simulink model "TorqueControl_QuadRad_FF_SMC"  (R2014a)
settings: Solver=ode4  StartTime=0.0  StopTime=4500  FixedStep=1  MaxStep=1  MinStep=0.1  RelTol=1e-3
undefined symbols (not defined in the file): bike, cont, param, paramIH, rider, route, sigbuilder_block
libraries: simulink x1, aerolibconvert2 x1
settings Model: Creator=Daniel  LastModifiedBy=meyer
settings SolverCC: InitialStep=1

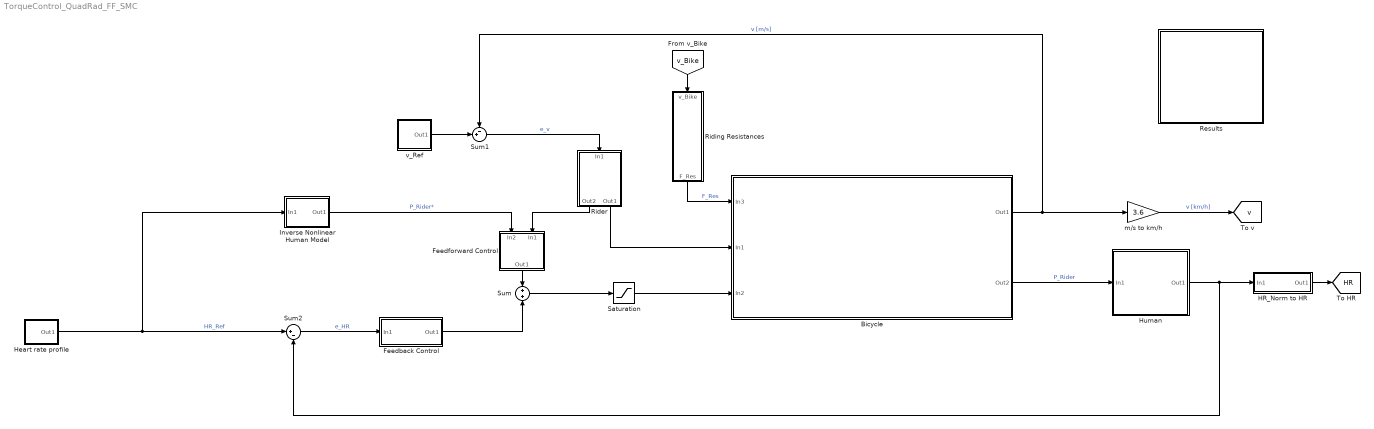
== system TorqueControl_QuadRad_FF_SMC ==
  Bicycle : Subsystem  mask(Bicycle Dynamics){}
      mask help:
      | Calculates the speed of the bicycle based on the propulsion forces of motor
      | bicycle rider against the resistance forces of the environment.
      mask Display:
      | port_label('input',1,'F_Res [N]')
      | port_label('input',2,'F_Rider [N]')
      | port_label('input',3,'T_M_ref')
      | port_label('output',1,'v_Bike [m/s]')
      | port_label('output',2,'P_Rider [W]')
      | image('QuadRad.jpg', [100 20 185 160])
  Feedback Control : Subsystem
  Feedforward Control : Subsystem
  HR_Norm to HR : Subsystem
  Heart rate profile : Subsystem
  Human : Subsystem
  Inverse Nonlinear Human Model : Subsystem
  Results : Subsystem
  Rider : Subsystem
  Riding Resistances : Subsystem
  Saturation : Saturate  UpperLimit=bike.motor.T_max  LowerLimit=bike.motor.T_min  ZeroCross=off
  Sum : Sum  Inputs=+|+
  Sum1 : Sum  Inputs=-+|
  Sum2 : Sum  Inputs=|+-
  m/s to km/h : Gain  Gain=3.6
  v_Ref : Subsystem
  tag scope: HR=global, v=global
  wires:
  Bicycle/1(Out1) -> Sum1/1, m/s to km/h/1  "v [m/s]"
  Riding Resistances/1(F_Res) -> Bicycle/1(In3)  "F_Res"
  m/s to km/h/1 -> [v]  "v [km/h]"
  [v_Bike] -> Riding Resistances/1(v_Bike)
  Sum1/1 -> Rider/1(In1)  "e_v"
  Rider/2(Out1) -> Bicycle/2(In1)
  HR_Norm to HR/1(Out1) -> [HR]
  Human/1(Out1) -> HR_Norm to HR/1(In1), Sum2/2
  Bicycle/2(Out2) -> Human/1(In1)  "P_Rider"
  Sum2/1 -> Feedback Control/1(In1)  "e_HR"
  Heart rate profile/1(Out1) -> Inverse Nonlinear Human Model/1(In1), Sum2/1  "HR_Ref"
  v_Ref/1(Out1) -> Sum1/2
  Feedback Control/1(Out1) -> Sum/2
  Sum/1 -> Saturation/1
  Rider/1(Out2) -> Feedforward Control/2(In1)
  Inverse Nonlinear Human Model/1(Out1) -> Feedforward Control/1(In2)  "P_Rider*"
  Feedforward Control/1(Out1) -> Sum/1
  Saturation/1 -> Bicycle/3(In2)

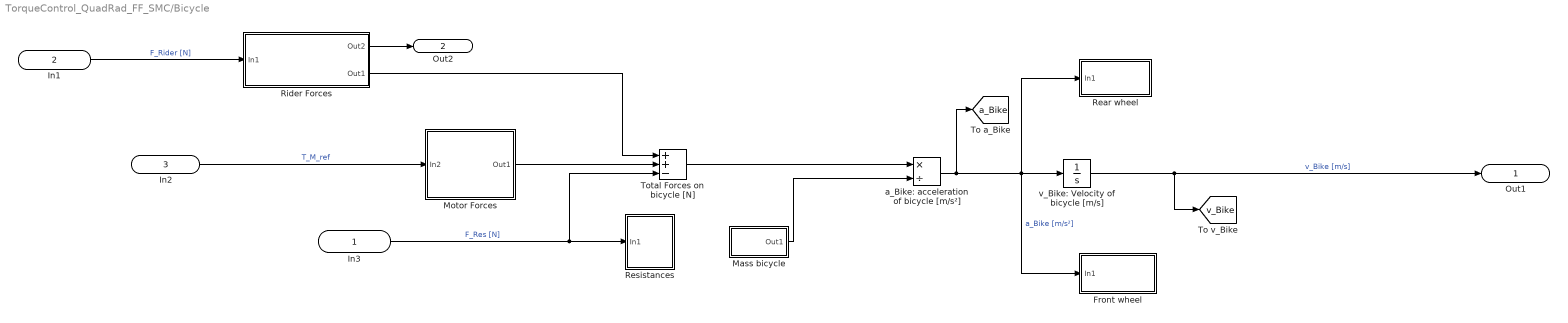
== system TorqueControl_QuadRad_FF_SMC/Bicycle ==
  In3 : Inport
  In1 : Inport  Port=2
  In2 : Inport  Port=3
  Front wheel : Subsystem
  Mass bicycle : Subsystem
  Motor Forces : Subsystem
  Rear wheel : Subsystem
  Resistances : Subsystem
  Rider Forces : Subsystem
  Total Forces on bicycle [N] : Sum  Inputs=++-
  a_Bike: acceleration of bicycle [m/s²] : Product  Inputs=*/
  v_Bike: Velocity of bicycle [m/s] : Integrator
  Out1 : Outport
  Out2 : Outport  Port=2
  tag scope: a_Bike=global, v_Bike=global
  wires:
  Mass bicycle/1(Out1) -> a_Bike: acceleration of bicycle [m/s²]/2
  Motor Forces/1(Out1) -> Total Forces on bicycle [N]/2
  In2/1 -> Motor Forces/1(In2)  "T_M_ref"
  Rider Forces/2(Out1) -> Total Forces on bicycle [N]/1
  Rider Forces/1(Out2) -> Out2/1
  In1/1 -> Rider Forces/1(In1)  "F_Rider [N]"
  a_Bike: acceleration of bicycle [m/s²]/1 -> v_Bike: Velocity of bicycle [m/s]/1, Rear wheel/1(In1), Front wheel/1(In1), [a_Bike]  "a_Bike [m/s²]"
  v_Bike: Velocity of bicycle [m/s]/1 -> Out1/1, [v_Bike]  "v_Bike [m/s]"
  Total Forces on bicycle [N]/1 -> a_Bike: acceleration of bicycle [m/s²]/1
  In3/1 -> Total Forces on bicycle [N]/3, Resistances/1(In1)  "F_Res [N]"

== system TorqueControl_QuadRad_FF_SMC/Feedback Control ==
  In1 : Inport
  Constant : Constant  Value=cont.c
  Derivative : Derivative
  Multiport Switch : MultiPortSwitch  Inputs=2
  Quasi-1-SMC : Subsystem
  Saturation : Saturate  UpperLimit=cont.upLim  LowerLimit=cont.lowLim
  Simple-1-SMC : Subsystem
  Out1 : Outport
  tag scope: T_M_FB=global, e=global, e_dot=global
  wires:
  Derivative/1 -> [e_dot]
  Quasi-1-SMC/1(Out1) -> Multiport Switch/3
  Simple-1-SMC/1(Out1) -> Multiport Switch/2
  Constant/1 -> Multiport Switch/1
  Saturation/1 -> [T_M_FB], Out1/1  "T_M_FB"
  In1/1 -> Simple-1-SMC/1(In1), Quasi-1-SMC/1(In1), [e], Derivative/1  "e_HR"
  Multiport Switch/1 -> Saturation/1  "T_M_FB"

== system TorqueControl_QuadRad_FF_SMC/Feedforward Control ==
  In2 : Inport
  In1 : Inport  Port=2
  Feedforward Control : Subsystem
  Sum3 : Sum  Inputs=-|+
  Out1 : Outport
  tag scope: T_M_FF=global
  wires:
  Feedforward Control/1(Out1) -> Sum3/1
  In2/1 -> Feedforward Control/1(In1)  "P_R*"
  In1/1 -> Sum3/2  "T_R"
  Sum3/1 -> Out1/1, [T_M_FF]  "T_M_FF"

== system TorqueControl_QuadRad_FF_SMC/HR_Norm to HR ==
  In1 : Inport
  Add : Sum
  HR_Rest : Constant  Value=rider.HR_rest
  HR_max : Constant  Value=rider.HR_max
  Product : Product
  Out1 : Outport
  wires:
  HR_max/1 -> Product/2
  Add/1 -> Out1/1  "HR"
  Product/1 -> Add/1
  In1/1 -> Product/1  "HR_Norm"
  HR_Rest/1 -> Add/2

== system TorqueControl_QuadRad_FF_SMC/Heart rate profile ==
  Choose HR_Profile : Constant  Value=3
  Constant : Constant  Value=140
  From Workspace : FromWorkspace  VariableName=HRPROFILE  SampleTime=0
  HR to HR_Norm : Subsystem
  Multiport Switch : MultiPortSwitch
  Signal Builder : Subsystem  Tag=STV Subsys  LoadFcn=sigbuilder_block('load');  StartFcn=sigbuilder_block('start');  StopFcn=sigbuilder_block('stop');  ClipboardFcn=sigbuilder_block('clipboard');  mask(Sigbuilder block){}
      mask help: Simulink:masks:SigbuilderBlock_MD
      mask init:
      | if ~strcmp(get_param(bdroot(gcbh),'SimulationStatus'),'stopped') tuvar = sigbuilder_block('maskInit'); end
      settings: CopyFcn=sigbuilder_block('copy');  DeleteFcn=sigbuilder_block('delete');  ModelCloseFcn=sigbuilder_block('modelClose');  PreSaveFcn=sigbuilder_block('preSave');  PauseFcn=sigbuilder_block('pause');  ContinueFcn=sigbuilder_block('continue');  NameChangeFcn=sigbuilder_block('namechange');  OpenFcn=sigbuilder_block('open',[216 88.5 550.5 394.5 ]);  CloseFcn=sigbuilder_block('close');
      mask Display: plot(0, 0, 100, 100,[2, 2, 32, 32, 2], [68, 8, 8, 68, 68],[32, 2], [38, 38], [32, 19, 2],[53, 60, 44], [32, 17, 17, 2],[16, 16, 31, 31]);txt = getActiveGroup(gcbh);text(2, 100, txt,'verticalAlignment', 'top');
  Out1 : Outport
  tag scope: HR_Ref=global, HR_Ref_Norm=global
  wires:
  Multiport Switch/1 -> HR to HR_Norm/1(In1), [HR_Ref]  "HRRef"
  HR to HR_Norm/1(Out1) -> [HR_Ref_Norm], Out1/1  "HR_Ref"
  Signal Builder/1(Signal 1) -> Multiport Switch/3  "HRRef"
  Constant/1 -> Multiport Switch/2
  Choose HR_Profile/1 -> Multiport Switch/1
  From Workspace/1 -> Multiport Switch/4

== system TorqueControl_QuadRad_FF_SMC/Human ==
  In1 : Inport
  Nonlinear Human Model : Subsystem
  Power to Power_Norm : Subsystem
  Scopex2 : Scope
      settings: SaveName=ScopeData2
  Out1 : Outport
  tag scope: x1=global, x2=global
  wires:
  In1/1 -> Power to Power_Norm/1(In1)  "P_Rider"
  Nonlinear Human Model/1(Out1) -> [x1], Out1/1  "Heart rate"
  Nonlinear Human Model/2(Out2) -> [x2], Scopex2/1
  Power to Power_Norm/1(Out1) -> Nonlinear Human Model/1(In1)

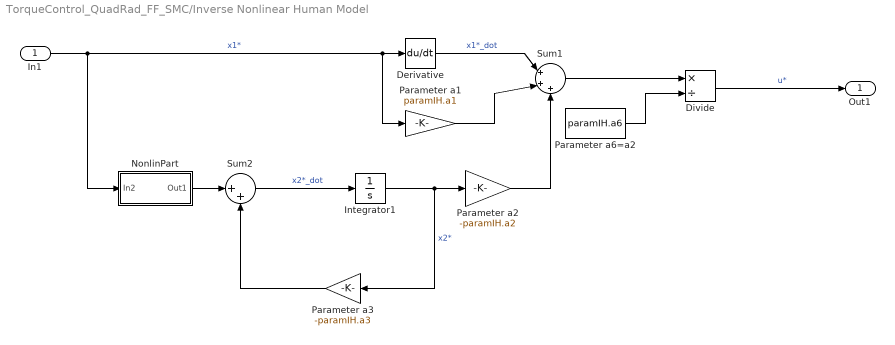
== system TorqueControl_QuadRad_FF_SMC/Inverse Nonlinear Human Model ==
  In1 : Inport
  Derivative : Derivative
  Divide : Product  Inputs=*/
  Integrator1 : Integrator
  NonlinPart : Subsystem
  Parameter a1 : Gain  Gain=paramIH.a1
  Parameter a2 : Gain  Gain=-paramIH.a2
  Parameter a3 : Gain  Gain=-paramIH.a3
  Parameter a6=a2 : Constant  Value=paramIH.a6
  Sum1 : Sum  Inputs=|+++
  Sum2 : Sum  Inputs=|++
  Out1 : Outport
  wires:
  Parameter a2/1 -> Sum1/3
  In1/1 -> Parameter a1/1, Derivative/1, NonlinPart/1(In2)  "x1*"
  Parameter a3/1 -> Sum2/2
  Sum2/1 -> Integrator1/1  "x2*_dot"
  Derivative/1 -> Sum1/1  "x1*_dot"
  Parameter a1/1 -> Sum1/2
  Sum1/1 -> Divide/1
  Parameter a6=a2/1 -> Divide/2
  Divide/1 -> Out1/1  "u*"
  NonlinPart/1(Out1) -> Sum2/1
  Integrator1/1 -> Parameter a3/1, Parameter a2/1  "x2*"

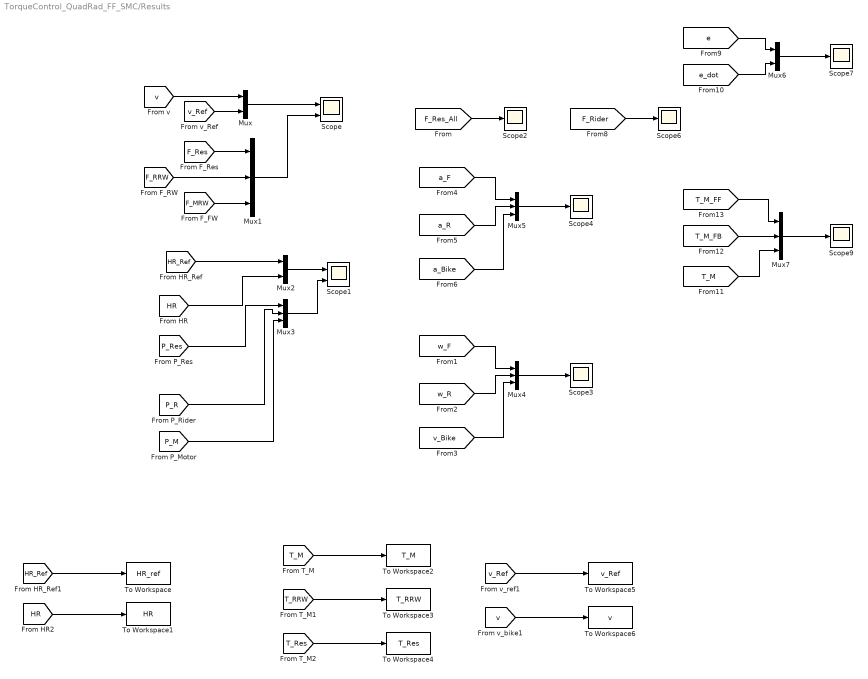
== system TorqueControl_QuadRad_FF_SMC/Results ==
  Mux : Mux  Inputs=2
  Mux{1,3..5,7} (5 alike) : Mux  Inputs=3
  Mux2 : Mux  Inputs=2
  Mux6 : Mux  Inputs=2
  Scope : Scope  NumInputPorts=2
      settings: TimeRange=4500  YMin=0~-50  YMax=25~200
  Scope1 : Scope  NumInputPorts=2
      settings: TimeRange=4500  YMin=75~0  YMax=155~375
  Scope{2..4,6..7,9} (6 alike) : Scope
      Scope2 settings: SaveName=ScopeData3
      Scope3 settings: SaveName=ScopeData4
      Scope4 settings: SaveName=ScopeData5
      Scope6 settings: SaveName=ScopeData7
      Scope7 settings: SaveName=ScopeData8
      Scope9 settings: SaveName=ScopeData10
  To Workspace : ToWorkspace  VariableName=HR_ref  SaveFormat=Timeseries  SampleTime=-1
  To Workspace1 : ToWorkspace  VariableName=HR  SaveFormat=Timeseries  SampleTime=-1
  To Workspace2 : ToWorkspace  VariableName=T_M  SaveFormat=Timeseries  SampleTime=-1
  To Workspace3 : ToWorkspace  VariableName=T_RRW  SaveFormat=Timeseries  SampleTime=-1
  To Workspace4 : ToWorkspace  VariableName=T_Res  SaveFormat=Timeseries  SampleTime=-1
  To Workspace5 : ToWorkspace  VariableName=v_Ref  SaveFormat=Timeseries  SampleTime=-1
  To Workspace6 : ToWorkspace  VariableName=v  SaveFormat=Timeseries  SampleTime=-1
  wires:
  [v] -> Mux/1
  [v_Ref] -> Mux/2
  Mux/1 -> Scope/1
  [F_Res] -> Mux1/1
  [F_MRW] -> Mux1/3
  Mux1/1 -> Scope/2
  [F_RRW] -> Mux1/2
  [HR_Ref] -> Mux2/1
  [HR] -> Mux2/2
  Mux2/1 -> Scope1/1
  [P_R] -> Mux3/2
  Mux3/1 -> Scope1/2
  [P_M] -> Mux3/3
  [P_Res] -> Mux3/1
  [F_Res_All] -> Scope2/1
  [w_F] -> Mux4/1
  [w_R] -> Mux4/2
  [v_Bike] -> Mux4/3
  Mux4/1 -> Scope3/1
  [a_F] -> Mux5/1
  [a_R] -> Mux5/2
  [a_Bike] -> Mux5/3
  Mux5/1 -> Scope4/1
  [F_Rider] -> Scope6/1
  Mux6/1 -> Scope7/1
  [e] -> Mux6/1
  [e_dot] -> Mux6/2
  [T_M] -> Mux7/3
  Mux7/1 -> Scope9/1
  [T_M_FF] -> Mux7/1
  [T_M_FB] -> Mux7/2
  [HR_Ref] -> To Workspace/1
  [HR] -> To Workspace1/1
  [T_M] -> To Workspace2/1
  [T_RRW] -> To Workspace3/1
  [T_Res] -> To Workspace4/1
  [v_Ref] -> To Workspace5/1
  [v] -> To Workspace6/1

== system TorqueControl_QuadRad_FF_SMC/Rider ==
  In1 : Inport
  Human Con : simulink/Continuous/PID Controller  Controller=PID  TimeDomain=Continuous-time  SampleTime=1  IntegratorMethod=Forward Euler  FilterMethod=Forward Euler  Form=Parallel  P=100  I=10  D=0  N=0  InitialConditionSource=internal  InitialConditionForIntegrator=0  InitialConditionForFilter=0  ExternalReset=none  LimitOutput=on  UpperSaturationLimit=900  LowerSaturationLimit=0  LinearizeAsGain=on  AntiWindupMode=none  Kb=1  TrackingMode=off  Kt=1  PParamMin=[]  PParamMax=[]  IParamMin=[]  IParamMax=[]  DParamMin=[]  DParamMax=[]  NParamMin=[]  NParamMax=[]  KbParamMin=[]  KbParamMax=[]  KtParamMin=[]  KtParamMax=[]  POutMin=[]  POutMax=[]  IOutMin=[]  IOutMax=[]  DOutMin=[]  DOutMax=[]  NOutMin=[]  NOutMax=[]  KbOutMin=[]  KbOutMax=[]  KtOutMin=[]  KtOutMax=[]  IntegratorOutMin=[]  IntegratorOutMax=[]  FilterOutMin=[]  FilterOutMax=[]  SumOutMin=[]  SumOutMax=[]  SumI1OutMin=[]  SumI1OutMax=[]  SumI2OutMin=[]  SumI2OutMax=[]  SumI3OutMin=[]  SumI3OutMax=[]  SumDOutMin=[]  SumDOutMax=[]  SaturationOutMin=[]  SaturationOutMax=[]  IntegratorContinuousStateAttributes=''  IntegratorStateMustResolveToSignalObject=off  IntegratorRTWStateStorageClass=Auto  FilterContinuousStateAttributes=''  FilterStateMustResolveToSignalObject=off  FilterRTWStateStorageClass=Auto
  Limit F_Rider : Subsystem
  Product1 : Product
  Saturation : Saturate  UpperLimit=900  LowerLimit=0
  r_C: crank length [m] : Constant  Value=bike.r_C
  tau: transmission ratio [-] : Constant  Value=bike.tau
  Out2 : Outport
  Out1 : Outport  Port=2
  tag scope: F_Rider=global
  wires:
  In1/1 -> Human Con/1  "e_v"
  Human Con/1 -> Limit F_Rider/1(In1), [F_Rider]  "F_Rider"
  r_C: crank length [m]/1 -> Product1/2, Limit F_Rider/3(In3)
  Product1/1 -> Out2/1  "T_Rider"
  Limit F_Rider/1(Out1) -> Saturation/1
  Saturation/1 -> Product1/1, Out1/1  "F_Rider"
  tau: transmission ratio [-]/1 -> Limit F_Rider/2(In2)

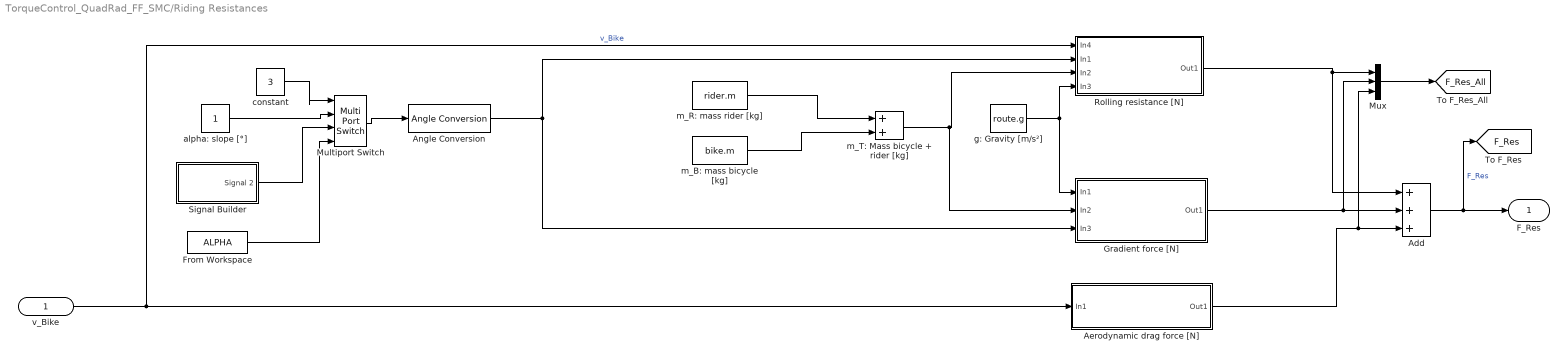
== system TorqueControl_QuadRad_FF_SMC/Riding Resistances ==
  v_Bike : Inport
  Add : Sum  Inputs=+++
  Aerodynamic drag force [N] : Subsystem
  Angle Conversion : aerolibconvert2/Angle Conversion  IU=deg  OU=rad
  From Workspace : FromWorkspace  VariableName=ALPHA  SampleTime=0
  Gradient force [N] : Subsystem
  Multiport Switch : MultiPortSwitch
  Mux : Mux  Inputs=3
  Rolling resistance [N] : Subsystem
  Signal Builder : Subsystem  Tag=STV Subsys  LoadFcn=sigbuilder_block('load');  StartFcn=sigbuilder_block('start');  StopFcn=sigbuilder_block('stop');  ClipboardFcn=sigbuilder_block('clipboard');  mask(Sigbuilder block){}
      mask help: Simulink:masks:SigbuilderBlock_MD
      mask init:
      | if ~strcmp(get_param(bdroot(gcbh),'SimulationStatus'),'stopped') tuvar = sigbuilder_block('maskInit'); end
      settings: CopyFcn=sigbuilder_block('copy');  DeleteFcn=sigbuilder_block('delete');  ModelCloseFcn=sigbuilder_block('modelClose');  PreSaveFcn=sigbuilder_block('preSave');  PauseFcn=sigbuilder_block('pause');  ContinueFcn=sigbuilder_block('continue');  NameChangeFcn=sigbuilder_block('namechange');  OpenFcn=sigbuilder_block('open',[437.25 118.5 550.5 394.5 ]);  CloseFcn=sigbuilder_block('close');
      mask Display: plot(0, 0, 100, 100,[2, 2, 32, 32, 2], [68, 8, 8, 68, 68],[32, 2], [38, 38], [32, 19, 2],[53, 60, 44], [32, 17, 17, 2],[16, 16, 31, 31]);txt = getActiveGroup(gcbh);text(2, 100, txt,'verticalAlignment', 'top');
  alpha: slope [°] : Constant
  constant : Constant  Value=3
  g: Gravity [m/s²] : Constant  Value=route.g
  m_B: mass bicycle [kg] : Constant  Value=bike.m
  m_R: mass rider [kg] : Constant  Value=rider.m
  m_T: Mass bicycle + rider [kg] : Sum
  F_Res : Outport
  tag scope: F_Res=global, F_Res_All=global
  wires:
  Mux/1 -> [F_Res_All]
  Gradient force [N]/1(Out1) -> Add/2, Mux/2
  Rolling resistance [N]/1(Out1) -> Mux/1, Add/1
  Aerodynamic drag force [N]/1(Out1) -> Add/3, Mux/3
  v_Bike/1 -> Aerodynamic drag force [N]/1(In1), Rolling resistance [N]/1(In4)  "v_Bike"
  Angle Conversion/1 -> Gradient force [N]/3(In3), Rolling resistance [N]/2(In1)
  Add/1 -> F_Res/1, [F_Res]  "F_Res"
  g: Gravity [m/s²]/1 -> Rolling resistance [N]/4(In3), Gradient force [N]/1(In1)
  Multiport Switch/1 -> Angle Conversion/1
  Signal Builder/1(Signal 2) -> Multiport Switch/3
  alpha: slope [°]/1 -> Multiport Switch/2
  constant/1 -> Multiport Switch/1
  From Workspace/1 -> Multiport Switch/4
  m_T: Mass bicycle + rider [kg]/1 -> Gradient force [N]/2(In2), Rolling resistance [N]/3(In2)
  m_R: mass rider [kg]/1 -> m_T: Mass bicycle + rider [kg]/1
  m_B: mass bicycle [kg]/1 -> m_T: Mass bicycle + rider [kg]/2

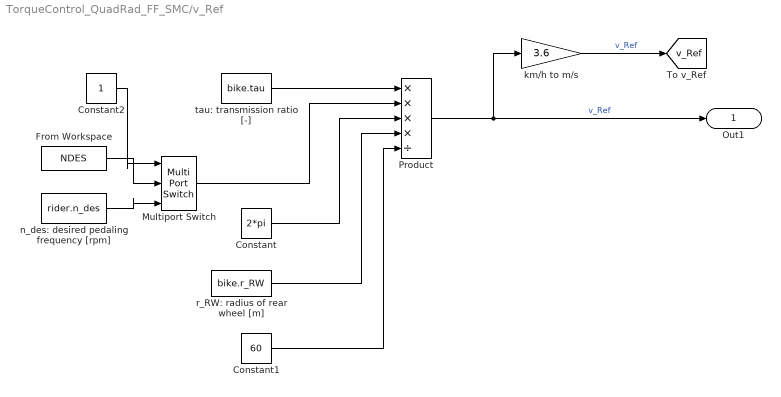
== system TorqueControl_QuadRad_FF_SMC/v_Ref ==
  Constant : Constant  Value=2*pi
  Constant1 : Constant  Value=60
  Constant2 : Constant
  From Workspace : FromWorkspace  VariableName=NDES  SampleTime=0
  Multiport Switch : MultiPortSwitch  Inputs=2
  Product : Product  Inputs=****/
  km/h to m/s : Gain  Gain=3.6
  n_des: desired pedaling frequency [rpm] : Constant  Value=rider.n_des
  r_RW: radius of rear wheel [m] : Constant  Value=bike.r_RW
  tau: transmission ratio [-] : Constant  Value=bike.tau
  Out1 : Outport
  tag scope: v_Ref=global
  wires:
  Product/1 -> km/h to m/s/1, Out1/1  "v_Ref"
  Constant/1 -> Product/3
  Constant1/1 -> Product/5
  km/h to m/s/1 -> [v_Ref]  "v_Ref"
  tau: transmission ratio [-]/1 -> Product/1
  r_RW: radius of rear wheel [m]/1 -> Product/4
  Multiport Switch/1 -> Product/2
  From Workspace/1 -> Multiport Switch/2
  n_des: desired pedaling frequency [rpm]/1 -> Multiport Switch/3
  Constant2/1 -> Multiport Switch/1

== system TorqueControl_QuadRad_FF_SMC/Bicycle/Front wheel ==
  In1 : Inport
  "a_F: angular acceleration of front wheel [rad/s²] " : Product  Inputs=*/
  r_FW: radius of front wheel [m] : Constant  Value=bike.r_FW
  w_F: angular velocity of front wheel [rad/s] : Integrator
  tag scope: a_F=global, w_F=global
  wires:
  w_F: angular velocity of front wheel [rad/s]/1 -> [w_F]
  "a_F: angular acceleration of front wheel [rad/s²] "/1 -> w_F: angular velocity of front wheel [rad/s]/1, [a_F]
  In1/1 -> "a_F: angular acceleration of front wheel [rad/s²] "/1  "a_Bike"
  r_FW: radius of front wheel [m]/1 -> "a_F: angular acceleration of front wheel [rad/s²] "/2

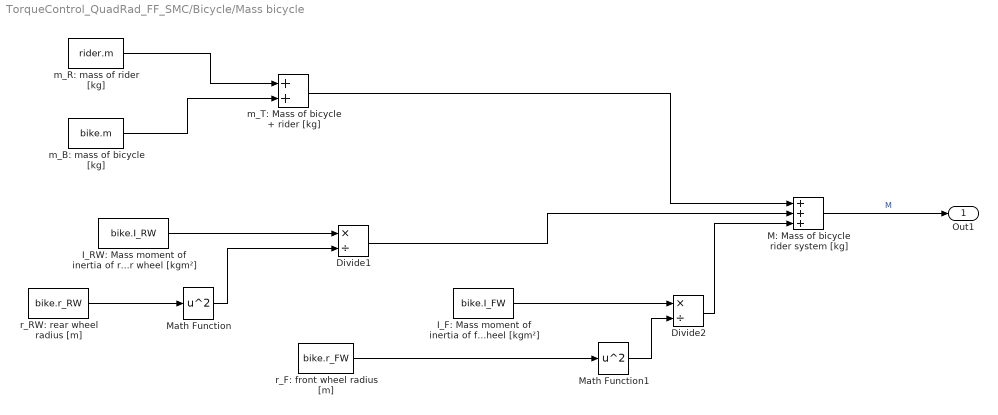
== system TorqueControl_QuadRad_FF_SMC/Bicycle/Mass bicycle ==
  Divide1 : Product  Inputs=*/
  Divide2 : Product  Inputs=*/
  I_F: Mass moment of inertia of front wheel [kgm²] : Constant  Value=bike.I_FW
  I_RW: Mass moment of inertia of rear wheel [kgm²] : Constant  Value=bike.I_RW
  M: Mass of bicycle rider system [kg] : Sum  Inputs=+++
  Math Function : Math  Operator=square  SaturateOnIntegerOverflow=on
  Math Function1 : Math  Operator=square  SaturateOnIntegerOverflow=on
  m_B: mass of bicycle [kg] : Constant  Value=bike.m
  m_R: mass of rider [kg] : Constant  Value=rider.m
  m_T: Mass of bicycle + rider [kg] : Sum
  r_F: front wheel radius [m] : Constant  Value=bike.r_FW
  r_RW: rear wheel radius [m] : Constant  Value=bike.r_RW
  Out1 : Outport
  wires:
  I_F: Mass moment of inertia of front wheel [kgm²]/1 -> Divide2/1
  Divide2/1 -> M: Mass of bicycle rider system [kg]/3
  M: Mass of bicycle rider system [kg]/1 -> Out1/1  "M"
  m_R: mass of rider [kg]/1 -> m_T: Mass of bicycle + rider [kg]/1
  r_RW: rear wheel radius [m]/1 -> Math Function/1
  Math Function/1 -> Divide1/2
  I_RW: Mass moment of inertia of rear wheel [kgm²]/1 -> Divide1/1
  Divide1/1 -> M: Mass of bicycle rider system [kg]/2
  r_F: front wheel radius [m]/1 -> Math Function1/1
  Math Function1/1 -> Divide2/2
  m_B: mass of bicycle [kg]/1 -> m_T: Mass of bicycle + rider [kg]/2
  m_T: Mass of bicycle + rider [kg]/1 -> M: Mass of bicycle rider system [kg]/1

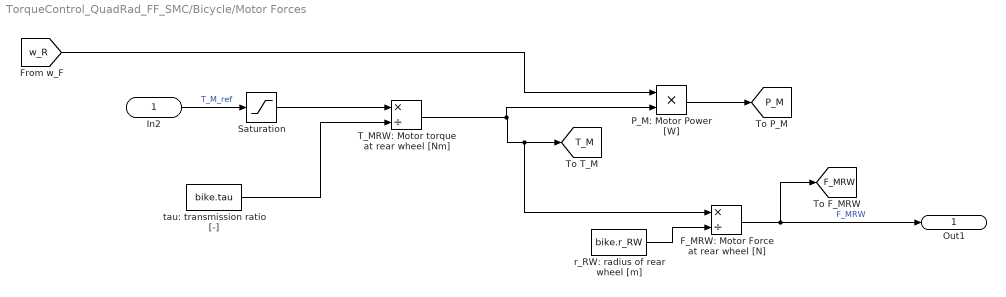
== system TorqueControl_QuadRad_FF_SMC/Bicycle/Motor Forces ==
  In2 : Inport
  F_MRW: Motor Force at rear wheel [N] : Product  Inputs=*/
  P_M: Motor Power [W] : Product  Inputs=**
  Saturation : Saturate  UpperLimit=bike.motor.T_max  LowerLimit=bike.motor.T_min  ZeroCross=off
  T_MRW: Motor torque at rear wheel [Nm] : Product  Inputs=*/
  r_RW: radius of rear wheel [m] : Constant  Value=bike.r_RW
  tau: transmission ratio [-] : Constant  Value=bike.tau
  Out1 : Outport
  tag scope: F_MRW=global, P_M=global, T_M=global
  wires:
  P_M: Motor Power [W]/1 -> [P_M]
  In2/1 -> Saturation/1  "T_M_ref"
  [w_R] -> P_M: Motor Power [W]/1
  F_MRW: Motor Force at rear wheel [N]/1 -> [F_MRW], Out1/1  "F_MRW"
  r_RW: radius of rear wheel [m]/1 -> F_MRW: Motor Force at rear wheel [N]/2
  Saturation/1 -> T_MRW: Motor torque at rear wheel [Nm]/1
  T_MRW: Motor torque at rear wheel [Nm]/1 -> P_M: Motor Power [W]/2, F_MRW: Motor Force at rear wheel [N]/1, [T_M]
  tau: transmission ratio [-]/1 -> T_MRW: Motor torque at rear wheel [Nm]/2

== system TorqueControl_QuadRad_FF_SMC/Bicycle/Rear wheel ==
  In1 : Inport
  "a_R: angular acceleration of rear wheel [rad/s²] " : Product  Inputs=/*
  r_RW: radius of rear wheel [m] : Constant  Value=bike.r_RW
  w_R: angular velocity of rear wheel [rad/s] : Integrator
  tag scope: a_R=global, w_R=global
  wires:
  "a_R: angular acceleration of rear wheel [rad/s²] "/1 -> w_R: angular velocity of rear wheel [rad/s]/1, [a_R]
  w_R: angular velocity of rear wheel [rad/s]/1 -> [w_R]
  In1/1 -> "a_R: angular acceleration of rear wheel [rad/s²] "/2  "a_Bike"
  r_RW: radius of rear wheel [m]/1 -> "a_R: angular acceleration of rear wheel [rad/s²] "/1

== system TorqueControl_QuadRad_FF_SMC/Bicycle/Resistances ==
  In1 : Inport
  P_Res: Riding resistances [W] : Product
  T_Res: Torque Riding resistances [Nm] : Product
  r_RW: radius of rear wheel [m] : Constant  Value=bike.r_RW
  tag scope: P_Res=global, T_Res=global
  wires:
  [w_R] -> P_Res: Riding resistances [W]/2
  P_Res: Riding resistances [W]/1 -> [P_Res]
  In1/1 -> T_Res: Torque Riding resistances [Nm]/1  "F_Res"
  T_Res: Torque Riding resistances [Nm]/1 -> [T_Res], P_Res: Riding resistances [W]/1
  r_RW: radius of rear wheel [m]/1 -> T_Res: Torque Riding resistances [Nm]/2

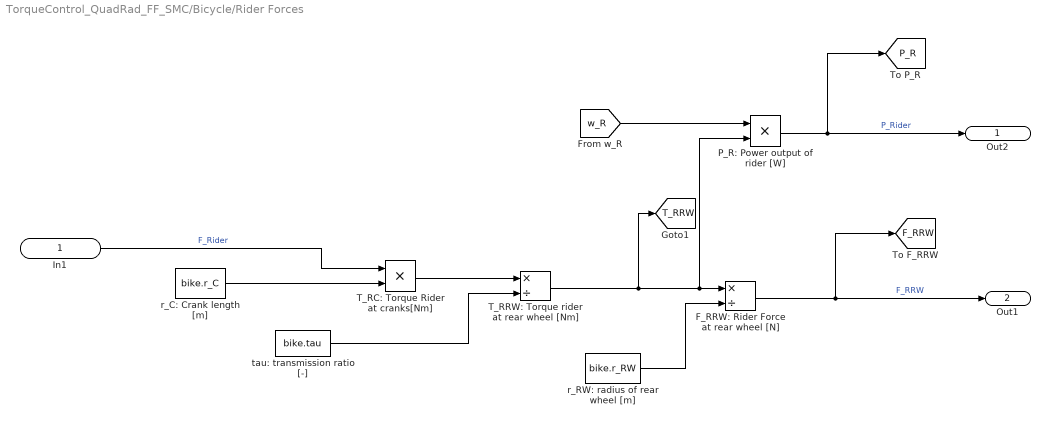
== system TorqueControl_QuadRad_FF_SMC/Bicycle/Rider Forces ==
  In1 : Inport
  F_RRW: Rider Force at rear wheel [N] : Product  Inputs=*/
  P_R: Power output of rider [W] : Product
  T_RC: Torque Rider at cranks[Nm] : Product
  T_RRW: Torque rider at rear wheel [Nm] : Product  Inputs=*/
  r_C: Crank length [m] : Constant  Value=bike.r_C
  r_RW: radius of rear wheel [m] : Constant  Value=bike.r_RW
  tau: transmission ratio [-] : Constant  Value=bike.tau
  Out2 : Outport
  Out1 : Outport  Port=2
  tag scope: F_RRW=global, P_R=global, T_RRW=global
  wires:
  F_RRW: Rider Force at rear wheel [N]/1 -> [F_RRW], Out1/1  "F_RRW"
  [w_R] -> P_R: Power output of rider [W]/1
  P_R: Power output of rider [W]/1 -> [P_R], Out2/1  "P_Rider"
  T_RC: Torque Rider at cranks[Nm]/1 -> T_RRW: Torque rider at rear wheel [Nm]/1
  r_C: Crank length [m]/1 -> T_RC: Torque Rider at cranks[Nm]/2
  T_RRW: Torque rider at rear wheel [Nm]/1 -> F_RRW: Rider Force at rear wheel [N]/1, P_R: Power output of rider [W]/2, [T_RRW]
  In1/1 -> T_RC: Torque Rider at cranks[Nm]/1  "F_Rider"
  tau: transmission ratio [-]/1 -> T_RRW: Torque rider at rear wheel [Nm]/2
  r_RW: radius of rear wheel [m]/1 -> F_RRW: Rider Force at rear wheel [N]/2

== system TorqueControl_QuadRad_FF_SMC/Feedback Control/Quasi-1-SMC ==
  In1 : Inport
  Sliding Surface : Subsystem
  Out1 : Outport
  wires:
  In1/1 -> Sliding Surface/1(In1)  "e_HR"
  Sliding Surface/1(Out1) -> Out1/1  "T_M_ref"

== system TorqueControl_QuadRad_FF_SMC/Feedback Control/Simple-1-SMC ==
  In1 : Inport
  Sliding Surface : Subsystem
  Out1 : Outport
  wires:
  In1/1 -> Sliding Surface/1(In1)  "e_HR"
  Sliding Surface/1(Out1) -> Out1/1  "T_M_ref"

== system TorqueControl_QuadRad_FF_SMC/Feedforward Control/Feedforward Control ==
  In1 : Inport
  Constant : Constant  Value=2*pi/60
  Power_Norm to Power1 : Subsystem
  Product : Product  Inputs=*/
  Product2 : Product
  n_des: desired pedaling frequency [rpm] : Constant  Value=rider.n_des
  Out1 : Outport
  wires:
  Product/1 -> Out1/1  "T_R*"
  Constant/1 -> Product2/2
  Product2/1 -> Product/2
  Power_Norm to Power1/1(Out1) -> Product/1
  In1/1 -> Power_Norm to Power1/1(In1)  "P_R*"
  n_des: desired pedaling frequency [rpm]/1 -> Product2/1

== system TorqueControl_QuadRad_FF_SMC/Heart rate profile/HR to HR_Norm ==
  In1 : Inport
  Divide : Product  Inputs=*/
  HR_Rest : Constant  Value=rider.HR_rest
  HR_max : Constant  Value=rider.HR_max
  Saturation : Saturate  UpperLimit=rider.HR_max  LowerLimit=rider.HR_rest
  Subtract : Sum  Inputs=+-
  Out1 : Outport
  wires:
  Subtract/1 -> Divide/1
  HR_max/1 -> Divide/2
  HR_Rest/1 -> Subtract/2
  Divide/1 -> Out1/1  "HR_Norm"
  In1/1 -> Saturation/1  "HR"
  Saturation/1 -> Subtract/1

== system TorqueControl_QuadRad_FF_SMC/Heart rate profile/Signal Builder ==
  Demux : Demux  Tag=STV Demux  Outputs=1
  FromWs : FromWorkspace  Tag=STV FromWs  VariableName=tuvar  SampleTime=0
      SigBuilderData=|
      | common.afterFinalStr = 'Extrapolate'
      | common.sampleTime = 0
      | dataSet.timeRange = [0 4500]
      | dataSet.name = 'Group 1'
      | sbobj.Groups.Name = 'Group 1'
      | sbobj.Groups.Signals.Name = 'Signal 1'
      | sbobj.Groups.Signals.XData = [0 200 1200 1400 2400 2600 3600 3800 4500]
      | sbobj.Groups.Signals.YData = [100 150 150 140 140 145 145 130 130]
      | sbobj.Groups.TimeRange = [0 4500]
  Signal 1 : Outport  Tag=STV Outport
  wires:
  FromWs/1 -> Demux/1
  Demux/1 -> Signal 1/1

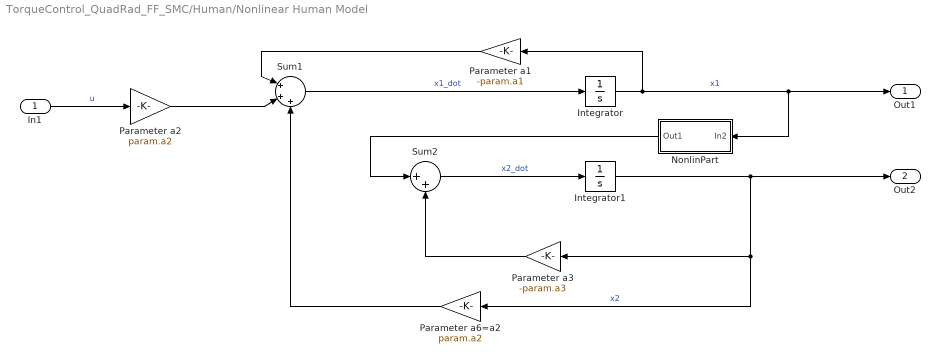
== system TorqueControl_QuadRad_FF_SMC/Human/Nonlinear Human Model ==
  In1 : Inport
  Integrator : Integrator
  Integrator1 : Integrator
  NonlinPart : Subsystem
  Parameter a1 : Gain  Gain=-param.a1
  Parameter a2 : Gain  Gain=param.a2
  Parameter a3 : Gain  Gain=-param.a3
  Parameter a6=a2 : Gain  Gain=param.a2
  Sum1 : Sum  Inputs=|+++
  Sum2 : Sum  Inputs=|++
  Out1 : Outport
  Out2 : Outport  Port=2
  wires:
  Integrator/1 -> Parameter a1/1, Out1/1, NonlinPart/1(In2)  "x1"
  Integrator1/1 -> Parameter a6=a2/1, Parameter a3/1, Out2/1  "x2"
  Parameter a6=a2/1 -> Sum1/3
  NonlinPart/1(Out1) -> Sum2/1
  Sum2/1 -> Integrator1/1  "x2_dot"
  Parameter a3/1 -> Sum2/2
  Parameter a1/1 -> Sum1/1
  In1/1 -> Parameter a2/1  "u"
  Sum1/1 -> Integrator/1  "x1_dot"
  Parameter a2/1 -> Sum1/2

== system TorqueControl_QuadRad_FF_SMC/Human/Power to Power_Norm ==
  In1 : Inport
  Constant : Constant  Value=rider.P_max
  Divide : Product  Inputs=*/
  Saturation : Saturate  UpperLimit=rider.P_max  LowerLimit=0  ZeroCross=off
  Out1 : Outport
  wires:
  Constant/1 -> Divide/2
  Divide/1 -> Out1/1  "Power_Norm"
  In1/1 -> Saturation/1  "Power"
  Saturation/1 -> Divide/1

== system TorqueControl_QuadRad_FF_SMC/Inverse Nonlinear Human Model/NonlinPart ==
  In2 : Inport
  Add : Sum
  Constant : Constant
  Divide1 : Product  Inputs=*/
  Math Function : Math  SaturateOnIntegerOverflow=on
  Parameter a4 : Gain  Gain=paramIH.a4
  Parameter a5 : Constant  Value=paramIH.a5
  Subtract : Sum  Inputs=-+
  Out1 : Outport
  wires:
  Subtract/1 -> Math Function/1
  Add/1 -> Divide1/2
  Math Function/1 -> Add/2
  Parameter a5/1 -> Subtract/2
  Constant/1 -> Add/1
  Divide1/1 -> Out1/1  "Nonlin"
  In2/1 -> Parameter a4/1, Subtract/1  "x1"
  Parameter a4/1 -> Divide1/1

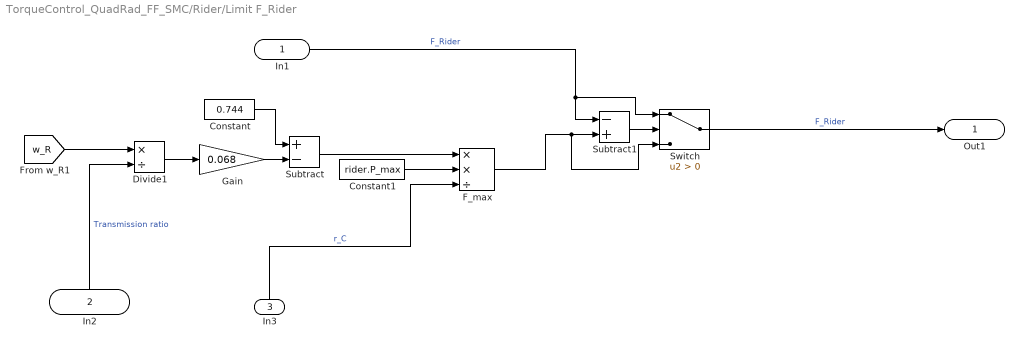
== system TorqueControl_QuadRad_FF_SMC/Rider/Limit F_Rider ==
  In1 : Inport
  In2 : Inport  Port=2
  In3 : Inport  Port=3
  Constant : Constant  Value=0.744
  Constant1 : Constant  Value=rider.P_max
  Divide1 : Product  Inputs=*/
  F_max : Product  Inputs=**/
  Gain : Gain  Gain=0.068
  Subtract : Sum  Inputs=+-
  Subtract1 : Sum  Inputs=-+
  Switch : Switch  Criteria=u2 > Threshold
  Out1 : Outport
  wires:
  Constant/1 -> Subtract/1
  Constant1/1 -> F_max/2
  [w_R] -> Divide1/1
  Divide1/1 -> Gain/1
  Switch/1 -> Out1/1  "F_Rider"
  Subtract1/1 -> Switch/2
  In3/1 -> F_max/3  "r_C"
  Subtract/1 -> F_max/1
  F_max/1 -> Subtract1/2, Switch/3
  In2/1 -> Divide1/2  "Transmission ratio"
  Gain/1 -> Subtract/2
  In1/1 -> Switch/1, Subtract1/1  "F_Rider"

== system TorqueControl_QuadRad_FF_SMC/Riding Resistances/Aerodynamic drag force [N] ==
  In1 : Inport
  A: Front Area [m²] : Constant  Value=bike.A
  Add1 : Sum
  F_Drag: Aerodynamical drag force [N] : Product  Inputs=5
  Factor : Constant  Value=0.5
  Math Function : Math  Operator=square  SaturateOnIntegerOverflow=on
  "c_w: Drag coefficient [-] " : Constant  Value=bike.cw
  roh: air density [kg/m³] : Constant  Value=1.25
  v_w: Headwind [m/s] : Constant  Value=route.v_w
  Out1 : Outport
  wires:
  Math Function/1 -> F_Drag: Aerodynamical drag force [N]/5
  v_w: Headwind [m/s]/1 -> Add1/2
  Add1/1 -> Math Function/1
  A: Front Area [m²]/1 -> F_Drag: Aerodynamical drag force [N]/4
  "c_w: Drag coefficient [-] "/1 -> F_Drag: Aerodynamical drag force [N]/3
  In1/1 -> Add1/1  "v_Bike [m/s]"
  Factor/1 -> F_Drag: Aerodynamical drag force [N]/2
  roh: air density [kg/m³]/1 -> F_Drag: Aerodynamical drag force [N]/1
  F_Drag: Aerodynamical drag force [N]/1 -> Out1/1  "F_Drag [N]"

== system TorqueControl_QuadRad_FF_SMC/Riding Resistances/Gradient force [N] ==
  In1 : Inport
  In2 : Inport  Port=2
  In3 : Inport  Port=3
  F_Slope: Gradient force [N] : Product  Inputs=3
  Trigonometric Function : Trigonometry
  Out1 : Outport
  wires:
  In1/1 -> F_Slope: Gradient force [N]/1  "g [m/s²]"
  In3/1 -> Trigonometric Function/1  "alpha [rad]"
  In2/1 -> F_Slope: Gradient force [N]/2  "m_T [kg]"
  Trigonometric Function/1 -> F_Slope: Gradient force [N]/3
  F_Slope: Gradient force [N]/1 -> Out1/1  "F_Slope [N]"

== system TorqueControl_QuadRad_FF_SMC/Riding Resistances/Rolling resistance [N] ==
  In4 : Inport
  In1 : Inport  Port=2
  In2 : Inport  Port=3
  In3 : Inport  Port=4
  Add : Sum
  F_DRoll: Dynamic Rolling resistance [N] : Product
  F_SRoll: Static Rolling resistance [N] : Product  Inputs=4
  Trigonometric Function1 : Trigonometry  Operator=cos
  f_DR: Dynamic Rolling resistance coefficient [Ns/m] : Constant  Value=bike.f_DR
  f_SR: Rolling resistance coefficient [-] : Constant  Value=bike.f_SR
  Out1 : Outport
  wires:
  Add/1 -> Out1/1  "F_Roll [N]"
  F_DRoll: Dynamic Rolling resistance [N]/1 -> Add/1
  In4/1 -> F_DRoll: Dynamic Rolling resistance [N]/2  "v_Bike [m/s]"
  f_DR: Dynamic Rolling resistance coefficient [Ns/m]/1 -> F_DRoll: Dynamic Rolling resistance [N]/1
  In1/1 -> Trigonometric Function1/1  "alpha [rad]"
  In3/1 -> F_SRoll: Static Rolling resistance [N]/4  "g [m/s²]"
  In2/1 -> F_SRoll: Static Rolling resistance [N]/3  "m_T [kg]"
  f_SR: Rolling resistance coefficient [-]/1 -> F_SRoll: Static Rolling resistance [N]/1
  Trigonometric Function1/1 -> F_SRoll: Static Rolling resistance [N]/2
  F_SRoll: Static Rolling resistance [N]/1 -> Add/2  "F_SRoll [N]"

== system TorqueControl_QuadRad_FF_SMC/Riding Resistances/Signal Builder ==
  Demux : Demux  Tag=STV Demux  Outputs=1
  FromWs : FromWorkspace  Tag=STV FromWs  VariableName=tuvar  SampleTime=0
      SigBuilderData=|
      | common.afterFinalStr = 'Extrapolate'
      | common.sampleTime = 0
      | dataSet.timeRange = [0 4500]
      | dataSet.name = 'Group 1'
      | sbobj.Groups.Name = 'Group 1'
      | sbobj.Groups.Signals.Name = 'Signal 2'
      | sbobj.Groups.Signals.XData = [0 200 200 1000 1000 2000 2000 3000 3000 4500]
      | sbobj.Groups.Signals.YData = [0.12 0.12 0.6 0.6 0.125 0.125 0.98 0.98 0.125 0.125]
      | sbobj.Groups.TimeRange = [0 4500]
  Signal 2 : Outport  Tag=STV Outport
  wires:
  FromWs/1 -> Demux/1
  Demux/1 -> Signal 2/1

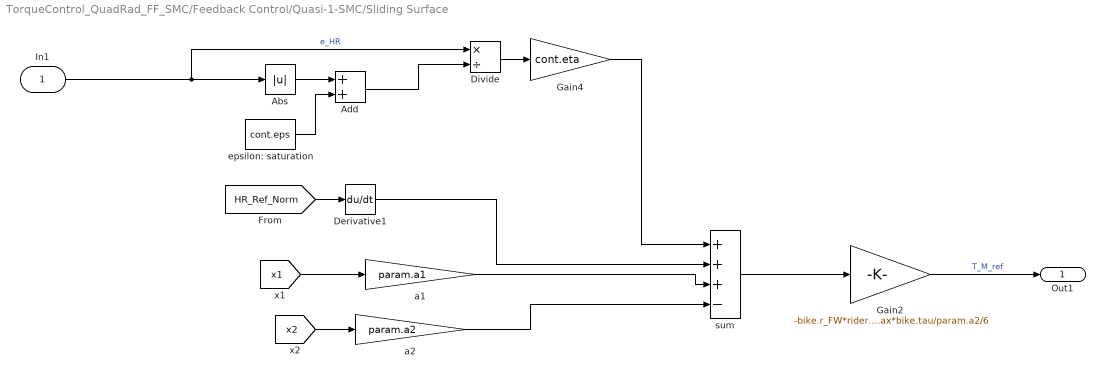
== system TorqueControl_QuadRad_FF_SMC/Feedback Control/Quasi-1-SMC/Sliding Surface ==
  In1 : Inport
  Abs : Abs  ZeroCross=off
  Add : Sum
  Derivative1 : Derivative
  Divide : Product  Inputs=*/
  Gain2 : Gain  Gain=-bike.r_FW*rider.P_max*bike.tau/param.a2/6
  Gain4 : Gain  Gain=cont.eta
  a1 : Gain  Gain=param.a1
  a2 : Gain  Gain=param.a2
  epsilon: saturation : Constant  Value=cont.eps  VectorParams1D=off
  sum : Sum  Inputs=+++-
  Out1 : Outport
  wires:
  Derivative1/1 -> sum/2
  In1/1 -> Divide/1, Abs/1  "e_HR"
  [x1] -> a1/1
  [HR_Ref_Norm] -> Derivative1/1
  a1/1 -> sum/3
  [x2] -> a2/1
  a2/1 -> sum/4
  sum/1 -> Gain2/1
  Divide/1 -> Gain4/1
  Gain2/1 -> Out1/1  "T_M_ref"
  Gain4/1 -> sum/1
  Abs/1 -> Add/1
  epsilon: saturation/1 -> Add/2
  Add/1 -> Divide/2

== system TorqueControl_QuadRad_FF_SMC/Feedback Control/Simple-1-SMC/Sliding Surface ==
  In1 : Inport
  Derivative1 : Derivative
  Gain2 : Gain  Gain=-bike.r_RW*rider.P_max*bike.tau/param.a2/6
  Gain4 : Gain  Gain=cont.eta
  Sign : Signum  ZeroCross=off
  a1 : Gain  Gain=param.a1
  a2 : Gain  Gain=param.a2
  sum : Sum  Inputs=+++-
  Out1 : Outport
  wires:
  Derivative1/1 -> sum/2
  In1/1 -> Sign/1  "e_HR"
  [x1] -> a1/1
  [HR_Ref_Norm] -> Derivative1/1
  a1/1 -> sum/3
  [x2] -> a2/1
  a2/1 -> sum/4
  sum/1 -> Gain2/1
  Sign/1 -> Gain4/1
  Gain2/1 -> Out1/1  "T_M_ref"
  Gain4/1 -> sum/1

== system TorqueControl_QuadRad_FF_SMC/Feedforward Control/Feedforward Control/Power_Norm to Power1 ==
  In1 : Inport
  P_max: maximum rider power [W] : Constant  Value=rider.P_max
  Product : Product
  Out1 : Outport
  wires:
  Product/1 -> Out1/1  "Power"
  In1/1 -> Product/1  "Power_Norm"
  P_max: maximum rider power [W]/1 -> Product/2

== system TorqueControl_QuadRad_FF_SMC/Human/Nonlinear Human Model/NonlinPart ==
  In2 : Inport
  Add : Sum
  Constant : Constant
  Divide1 : Product  Inputs=*/
  Math Function : Math  SaturateOnIntegerOverflow=on
  Parameter a4 : Gain  Gain=param.a4
  Parameter a5 : Constant  Value=param.a5
  Subtract : Sum  Inputs=-+
  Out1 : Outport
  wires:
  Parameter a4/1 -> Divide1/1
  In2/1 -> Subtract/1, Parameter a4/1  "x1"
  Divide1/1 -> Out1/1  "Nonlin"
  Constant/1 -> Add/1
  Parameter a5/1 -> Subtract/2
  Math Function/1 -> Add/2
  Add/1 -> Divide1/2
  Subtract/1 -> Math Function/1
